simulink model "sim_test_observer"  (Simulink 8.6)
settings: Solver=VariableStepAuto  StartTime=0.0  StopTime=100  RelTol=1e-3
libraries: cstblocks x4
settings Model: Creator=lbromo12  LastModifiedBy=lbromo12
settings DataIOCC: SaveFormat=Dataset  SignalLoggingSaveFormat=Dataset
settings OptimizationCC: ExpressionDepthLimit=128
settings DebuggingCC: UnderspecifiedInitializationDetection=Simplified  MergeDetectMultiDrivingBlocksExec=error  SolverPrmCheckMsg=none  FcnCallInpInsideContextMsg=EnableAllAsError  StateNameClashWarn=none
settings HardwareCC: ProdBitPerPointer=64  ProdLargestAtomicFloat=Float  ProdIntDivRoundTo=Zero  ProdEndianess=LittleEndian  ProdWordSize=64  ProdHWDeviceType=Intel->x86-64 (Windows64)
settings GRTTargetCC: GeneratePreprocessorConditionals=Use local settings  CombineOutputUpdateFcns=on  GRTInterface=off
settings ConfigComp: CovModelRefEnable=off

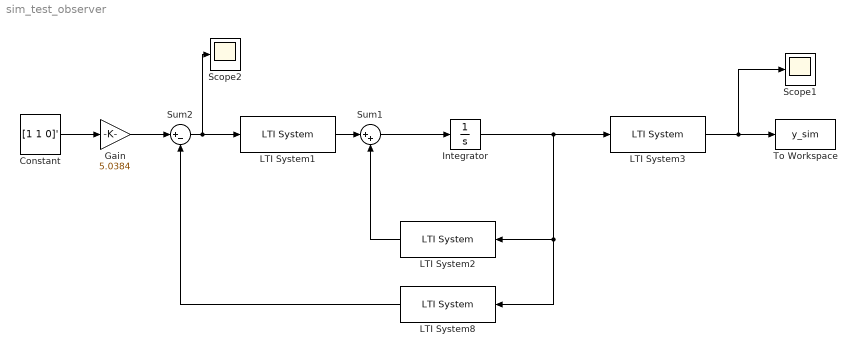
== system sim_test_observer ==
  Constant : Constant  Value=[1 1 0]'
  Gain : Gain  Gain=5.0384
  Integrator : Integrator
  LTI System1 : cstblocks/LTI System  sys=B  IC=[]
  LTI System2 : cstblocks/LTI System  sys=A  IC=[]
  LTI System3 : cstblocks/LTI System  sys=C  IC=[]
  LTI System8 : cstblocks/LTI System  sys=K  IC=[]
  Scope1 : Scope
  Scope2 : Scope
  Sum1 : Sum  Inputs=|++
  Sum2 : Sum  Inputs=|+-
  To Workspace : ToWorkspace  VariableName=y_sim  SaveFormat=Timeseries  SampleTime=-1
  wires:
  LTI System2/1 -> Sum1/2
  LTI System1/1 -> Sum1/1
  Sum1/1 -> Integrator/1
  LTI System3/1 -> Scope1/1, To Workspace/1
  Integrator/1 -> LTI System3/1, LTI System8/1, LTI System2/1
  Sum2/1 -> Scope2/1, LTI System1/1
  LTI System8/1 -> Sum2/2
  Constant/1 -> Gain/1
  Gain/1 -> Sum2/1
